simulink model "lab6"  (R2022b)
settings: Solver=VariableStepAuto  StartTime=0.0  StopTime=10.0  RelTol=1e-3
values from neighbouring files (symbols this model uses):
  Ts = 0.02    [ex1.m]    (also in lab07.m; s270874.mat)
libraries: cstblocks x2
settings Model: Creator=S270874  LastModifiedBy=franc
settings ModelReferenceCC: EnableRefExpFcnMdlSchedulingChecks=on

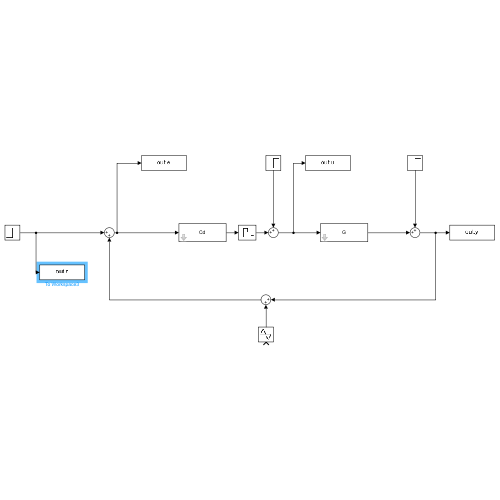
[thumbnail: Simulink's stored preview of the top-level diagram]
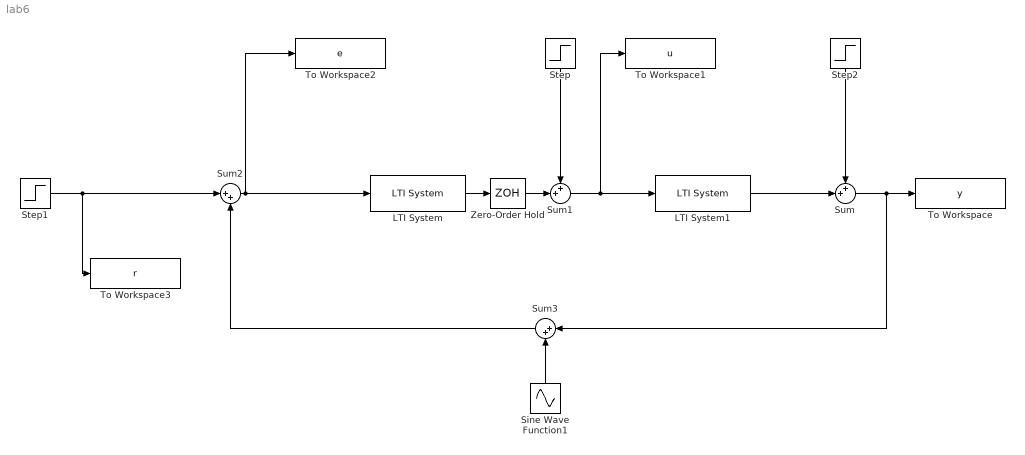
== system lab6 ==
  LTI System : cstblocks/LTI System  sys=Cd  IC=[]
  LTI System1 : cstblocks/LTI System  sys=G  IC=[]
  Sine Wave Function1 : Sin  TimeSource=Use external signal  SampleTime=0
  Step : Step  Time=0  SampleTime=0
  Step1 : Step  Time=0  SampleTime=0
  Step2 : Step  Time=0  SampleTime=0
  Sum : Sum  Inputs=++|
  Sum1 : Sum  Inputs=++|
  Sum2 : Sum  Inputs=|++
  Sum3 : Sum  Inputs=|++
  To Workspace : ToWorkspace  VariableName=y  SaveFormat=Timeseries  SampleTime=-1
  To Workspace1 : ToWorkspace  VariableName=u  SaveFormat=Timeseries  SampleTime=-1
  To Workspace2 : ToWorkspace  VariableName=e  SaveFormat=Timeseries  SampleTime=-1
  To Workspace3 : ToWorkspace  VariableName=r  SaveFormat=Timeseries  SampleTime=-1
  Zero-Order Hold : ZeroOrderHold  SampleTime=Ts
  wires:
  Step1/1 -> To Workspace3/1, Sum2/1
  Step/1 -> Sum1/1
  Sum1/1 -> To Workspace1/1, LTI System1/1
  Sum2/1 -> To Workspace2/1, LTI System/1
  Sum/1 -> Sum3/1, To Workspace/1
  LTI System/1 -> Zero-Order Hold/1
  Step2/1 -> Sum/1
  LTI System1/1 -> Sum/2
  Zero-Order Hold/1 -> Sum1/2
  Sine Wave Function1/1 -> Sum3/2
  Sum3/1 -> Sum2/2
